simulink model "ex4_dcmotor"  (R2025b)
settings: Solver=VariableStepAuto  StartTime=0.0  StopTime=0.1  RelTol=1e-3
values from neighbouring files (symbols this model uses):
  par = param_setter(0.23*10^(-3), 23.4*10^(-3), 2.4, 0.23*10^(-6), 0.4191*10^(-5))    [model_runner.m]
settings Model: Creator=fred  LastModifiedBy=fred

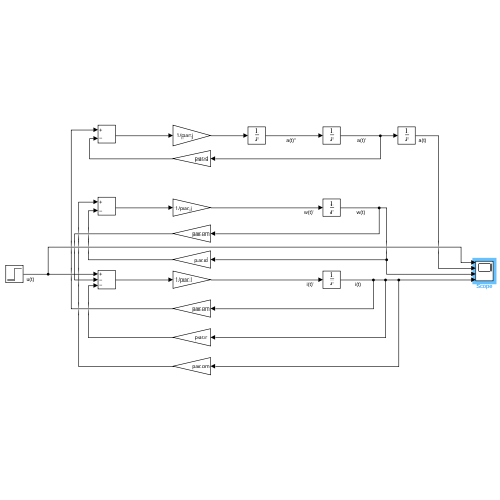
[thumbnail: Simulink's stored preview of the top-level diagram]
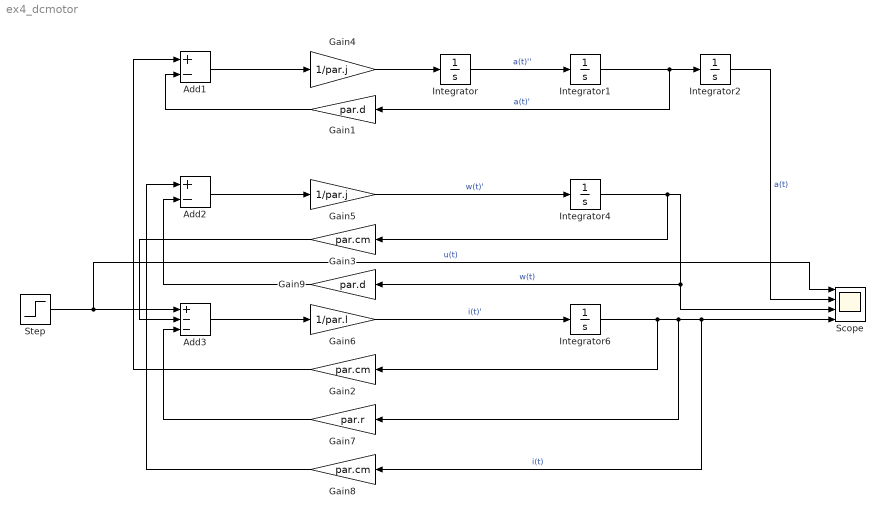
== system ex4_dcmotor ==
  Add1 : Sum  Inputs=+-
  Add2 : Sum  Inputs=+-
  Add3 : Sum  Inputs=+--
  Gain1 : Gain  Gain=par.d
  Gain2 : Gain  Gain=par.cm
  Gain3 : Gain  Gain=par.cm
  Gain4 : Gain  Gain=1/par.j
  Gain5 : Gain  Gain=1/par.j
  Gain6 : Gain  Gain=1/par.l
  Gain7 : Gain  Gain=par.r
  Gain8 : Gain  Gain=par.cm
  Gain9 : Gain  Gain=par.d
  Integrator{,1..2,4,6} (5 alike) : Integrator
  Scope : Scope  NumInputPorts=4
      settings: ActiveDisplayYMinimum=-3.9135545761809496  ActiveDisplayYMaximum=5.6377521346134589  DataLoggingVariableName=output
  Step : Step  Time=0  SampleTime=0
  wires:
  Integrator1/1 -> Gain1/1, Integrator2/1  "a(t)'"
  Integrator/1 -> Integrator1/1  "a(t)''"
  Integrator2/1 -> Scope/2  "a(t)"
  Integrator4/1 -> Scope/3, Gain9/1, Gain3/1  "w(t)"
  Gain6/1 -> Integrator6/1  "i(t)'"
  Integrator6/1 -> Gain2/1, Gain8/1, Scope/4, Gain7/1  "i(t)"
  Gain1/1 -> Add1/2
  Gain2/1 -> Add1/1
  Add1/1 -> Gain4/1
  Gain4/1 -> Integrator/1
  Add2/1 -> Gain5/1
  Add3/1 -> Gain6/1
  Step/1 -> Scope/1, Add3/1  "u(t)"
  Gain7/1 -> Add3/3
  Gain3/1 -> Add3/2
  Gain8/1 -> Add2/1
  Gain9/1 -> Add2/2
  Gain5/1 -> Integrator4/1  "w(t)'"
